simulink model "Model_6"  (R2020b)
settings: Solver=VariableStepAuto  StartTime=0.0  StopTime=10.0  RelTol=1e-3
settings Model: Creator=Akarsh  LastModifiedBy=Akarsh

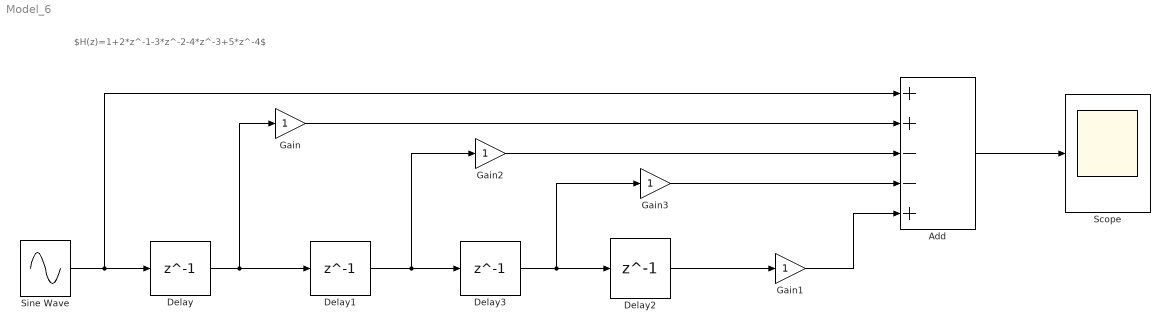
== system Model_6 ==
  note: $H(z)=1+2*z^-1-3*z^-2-4*z^-3+5*z^-4$
  Add : Sum  Inputs=++--+
  Delay{,1..3} (4 alike) : Delay  DelayLength=1
  Gain{,1..3} (4 alike) : Gain
  Scope : Scope
  Sine Wave : Sin  SampleTime=0
  wires:
  Delay/1 -> Gain/1, Delay1/1
  Delay1/1 -> Gain2/1, Delay3/1
  Delay3/1 -> Gain3/1, Delay2/1
  Delay2/1 -> Gain1/1
  Add/1 -> Scope/1
  Sine Wave/1 -> Add/1, Delay/1
  Gain/1 -> Add/2
  Gain2/1 -> Add/3
  Gain3/1 -> Add/4
  Gain1/1 -> Add/5
